simulink model "Trigonometric"  (R2020a)
settings: Solver=VariableStepAuto  StartTime=0.0  StopTime=10.0  RelTol=1e-3
settings Model: Creator=Mohammad  LastModifiedBy=Mohammad

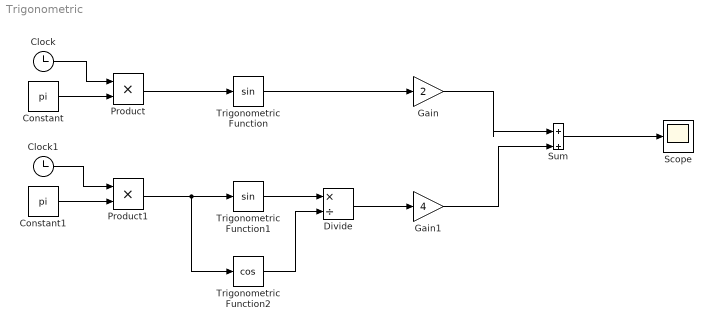
== system Trigonometric ==
  Clock : Clock
  Clock1 : Clock
  Constant : Constant  Value=pi
  Constant1 : Constant  Value=pi
  Divide : Product  Inputs=*/
  Gain : Gain  Gain=2
  Gain1 : Gain  Gain=4
  Product : Product
  Product1 : Product
  Scope : Scope
  Sum : Sum  Inputs=|++
  Trigonometric Function : Trigonometry
  Trigonometric Function1 : Trigonometry
  Trigonometric Function2 : Trigonometry  Operator=cos
  wires:
  Gain1/1 -> Sum/2
  Gain/1 -> Sum/1
  Trigonometric Function/1 -> Gain/1
  Constant1/1 -> Product1/2
  Clock1/1 -> Product1/1
  Constant/1 -> Product/2
  Clock/1 -> Product/1
  Product/1 -> Trigonometric Function/1
  Product1/1 -> Trigonometric Function2/1, Trigonometric Function1/1
  Divide/1 -> Gain1/1
  Trigonometric Function1/1 -> Divide/1
  Trigonometric Function2/1 -> Divide/2
  Sum/1 -> Scope/1
